simulink model "blockDiagramTask1"  (R2025a)
settings: Solver=VariableStepAuto  StartTime=0.0  StopTime=1  RelTol=1e-3
InitFcn:
  | run motor_specs.m
model workspace: external: MATLAB File C:\Users\josef\Desktop\KTH\MF2030\task1\motor_specs.m (data not in the file)
values from neighbouring files (symbols this model uses):
  A = [(-R/L), (-K_E/L); K_M/J, (-C_V/J)]    [ssAndTF.m]
  B = [(1/L), 0; 0, (-1/J)]    [ssAndTF.m]
  C = [1, 0; 0, 1]    [ssAndTF.m]
  D = zeros(2,2)    [ssAndTF.m]
undefined symbols (not defined in the file or in its folder): C_V, J, K_E, K_M, L, R, U_N
settings Model: Creator=josef  LastModifiedBy=josef

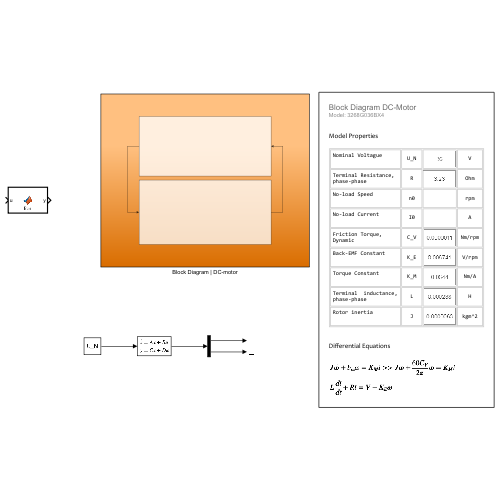
[thumbnail: Simulink's stored preview of the top-level diagram]
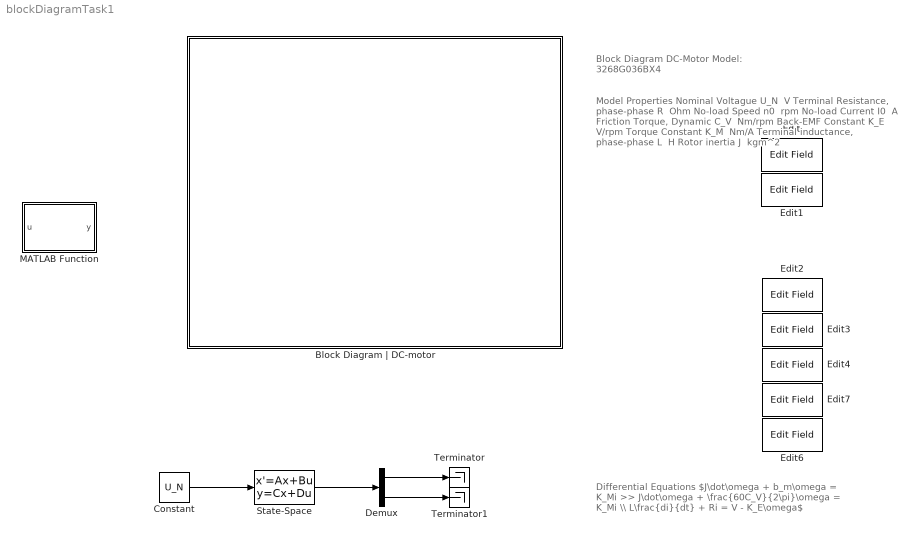
== system blockDiagramTask1 ==
  note: Differential Equations
      |
      | $J\dot\omega + b_m\omega = K_Mi >> J\dot\omega + \frac{60C_V}{2\pi}\omega = K_Mi \\ L\frac{di}{dt} + Ri = V - K_E\omega$
  note: Model Properties
      |
      | Nominal Voltague
      |
      | U_N
      | ​
      | V
      |
      | Terminal Resistance,
      | phase-phase
      | R
      | ​
      | Ohm
      |
      | No-load Speed
      |
      | n0
      | ​
      | rpm
      |
      | No-load Current
      |
      | I0
      | ​
      | A
      |
      | Friction Torque,
      | Dynamic
      | C_V
      | ​
      | Nm/rpm
      |
      | Back-EMF Constant
      |
      | K_E
      | ​
      | V/rpm
      |
      | Torque Constant
      |
      | K_M
      | ​
      | Nm/A
      |
      | Terminal inductance,
      | phase-phase
      | L
      | ​
      | H
      |
      | Rotor inertia
      |
      | J
      | ​
      | kgm^2
  note: Block Diagram DC-Motor
      | Model: 3268G036BX4
  Block Diagram | DC-motor : Subsystem
  Constant : Constant  Value=U_N
  Demux : Demux  Outputs=2
  Edit{,1..4,6..7} (7 alike) : EditField  LabelPosition=Hide  ShowInitialText=on  Alignment=Center  Opacity=0
  MATLAB Function : MATLAB Function  TreatAsAtomicUnit=on
  State-Space : StateSpace  A=A  B=B  C=C  D=D  InitialCondition=0
  Terminator : Terminator
  Terminator1 : Terminator
  wires:
  Constant/1 -> State-Space/1
  State-Space/1 -> Demux/1
  Demux/1 -> Terminator/1
  Demux/2 -> Terminator1/1

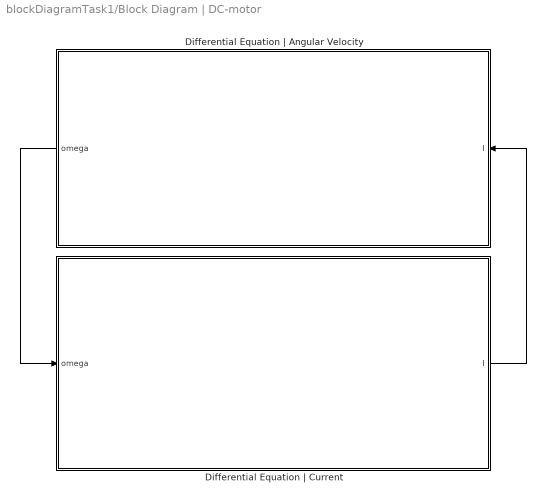
== system blockDiagramTask1/Block Diagram | DC-motor ==
  Differential Equation | Angular Velocity : Subsystem
  Differential Equation | Current : Subsystem
  wires:
  Differential Equation | Current/1(I) -> Differential Equation | Angular Velocity/1(I)
  Differential Equation | Angular Velocity/1(omega) -> Differential Equation | Current/1(omega)

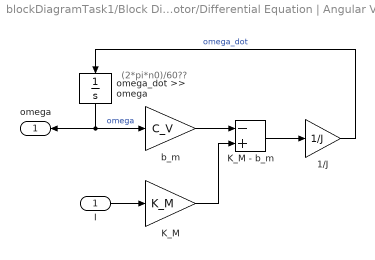
== system blockDiagramTask1/Block Diagram | DC-motor/Differential Equation | Angular Velocity ==
  note: (2*pi*n0)/60??
  I : Inport
  1/J : Gain  Gain=1/J
  K_M : Gain  Gain=K_M
  K_M - b_m : Sum  Inputs=-+
  b_m : Gain  Gain=C_V
  omega_dot >> omega : Integrator
  omega : Outport
  wires:
  b_m/1 -> K_M - b_m/1
  omega_dot >> omega/1 -> omega/1, b_m/1  "omega"
  K_M/1 -> K_M - b_m/2
  K_M - b_m/1 -> 1/J/1
  I/1 -> K_M/1
  1/J/1 -> omega_dot >> omega/1  "omega_dot"

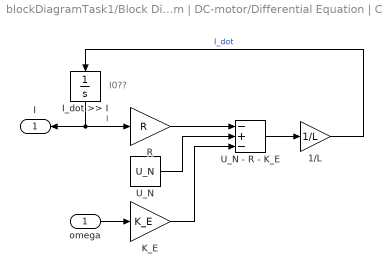
== system blockDiagramTask1/Block Diagram | DC-motor/Differential Equation | Current ==
  note: I0??
  omega : Inport
  1/L : Gain  Gain=1/L
  I_dot >> I : Integrator
  K_E : Gain  Gain=K_E
  R : Gain  Gain=R
  U_N : Constant  Value=U_N
  U_N - R - K_E : Sum  Inputs=-+-
  I : Outport
  wires:
  I_dot >> I/1 -> R/1, I/1  "I"
  K_E/1 -> U_N - R - K_E/3
  U_N - R - K_E/1 -> 1/L/1
  omega/1 -> K_E/1
  R/1 -> U_N - R - K_E/1
  1/L/1 -> I_dot >> I/1  "I_dot"
  U_N/1 -> U_N - R - K_E/2

== matlab function blockDiagramTask1/MATLAB Function ==
  data: u input; y output
function y = fcn(u)

y = u;
